simulink model "homework5"  (R2014b)
settings: Solver=ode45  SolverMode=SingleTasking  StartTime=0.0  StopTime=10.0  RelTol=1e-3
values from neighbouring files (symbols this model uses):
  A = [[      Y_v,       Y_p,    Y_r - u_0, g * cos(theta_0), 0] ... (first row only)    [hw5.m]
  B = [Y_d_r       Y_d_a ... (first row only)    [hw5.m]
  C = [[1/u_0, 0, 0, 0, 0] ... (first row only)    [hw5.m]
  D = [0 0 ... (first row only)    [hw5.m]
  g = 32.2    [hw5.m]
  u_0 = 468.2    [hw5.m]
settings Model: CovSFcnEnable=on  Creator=karasinski  LastModifiedBy=karasinski
settings OptimizationCC: BlockReduction=off  BooleanDataType=off
settings DebuggingCC: SaveWithParameterizedLinksMsg=none  UnderspecifiedInitializationDetection=Classic  MergeDetectMultiDrivingBlocksExec=none  SignalResolutionControl=TryResolveAllWithWarning  SolverPrmCheckMsg=none
settings HardwareCC: TargetUnknown=on

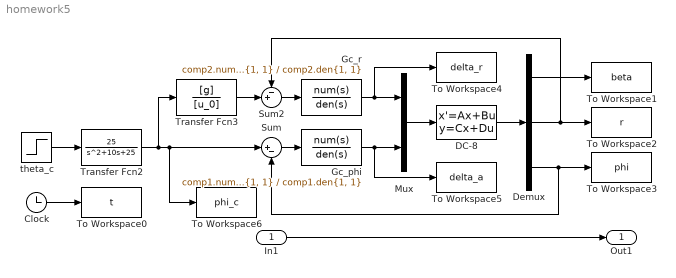
== system homework5 ==
  In1 : Inport
  Clock : Clock
  DC-8 : StateSpace  A=A  B=B  C=C  D=D  X0=0
  Demux : Demux  Outputs=3
  Gc_phi : TransferFcn  Numerator=comp1.num{1, 1}  Denominator=comp1.den{1, 1}
  Gc_r : TransferFcn  Numerator=comp2.num{1, 1}  Denominator=comp2.den{1, 1}
  Mux : Mux  Inputs=2
  Sum : Sum  Inputs=|+-
  Sum2 : Sum  Inputs=-+|
  To Workspace0 : ToWorkspace  VariableName=t  SampleTime=-1
  To Workspace1 : ToWorkspace  VariableName=beta  SampleTime=-1
  To Workspace2 : ToWorkspace  VariableName=r  SampleTime=-1
  To Workspace3 : ToWorkspace  VariableName=phi  SampleTime=-1
  To Workspace4 : ToWorkspace  VariableName=delta_r  SampleTime=-1
  To Workspace5 : ToWorkspace  VariableName=delta_a  SampleTime=-1
  To Workspace6 : ToWorkspace  VariableName=phi_c  SampleTime=-1
  Transfer Fcn2 : TransferFcn  Numerator=[25]  Denominator=[1 10 25]
  Transfer Fcn3 : TransferFcn  Numerator=[g]  Denominator=[u_0]
  theta_c : Step  Time=0  After=20 / 57.3  SampleTime=0
  Out1 : Outport
  wires:
  DC-8/1 -> Demux/1
  Mux/1 -> DC-8/1
  Demux/1 -> To Workspace1/1
  Demux/2 -> To Workspace2/1, Sum2/1
  Clock/1 -> To Workspace0/1
  Gc_r/1 -> Mux/1, To Workspace4/1
  Gc_phi/1 -> Mux/2, To Workspace5/1
  theta_c/1 -> Transfer Fcn2/1
  Transfer Fcn3/1 -> Sum2/2
  Transfer Fcn2/1 -> To Workspace6/1, Sum/1, Transfer Fcn3/1
  Demux/3 -> Sum/2, To Workspace3/1
  Sum/1 -> Gc_phi/1
  Sum2/1 -> Gc_r/1
  In1/1 -> Out1/1
